simulink model "SixteenMuxInput"  (R2024b)
settings: Solver=VariableStepAuto  StartTime=0.0  StopTime=10.0  RelTol=1e-3
settings Model: Creator=ferbe  LastModifiedBy=ferbe

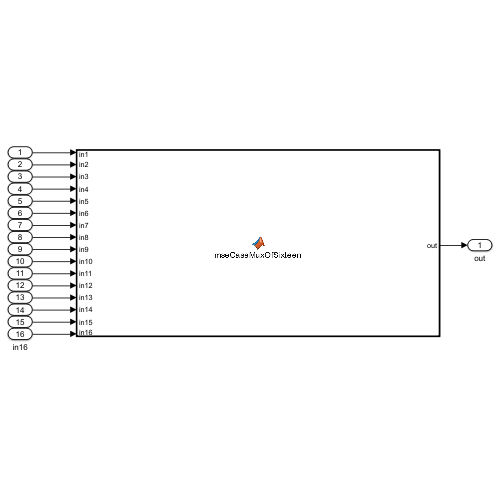
[thumbnail: Simulink's stored preview of the top-level diagram]
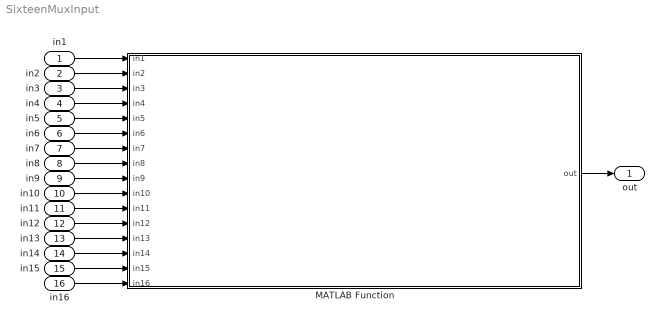
== system SixteenMuxInput ==
  in1 : Inport
  in2 : Inport  Port=2
  in3 : Inport  Port=3
  in4 : Inport  Port=4
  in5 : Inport  Port=5
  in6 : Inport  Port=6
  in7 : Inport  Port=7
  in8 : Inport  Port=8
  in9 : Inport  Port=9
  in10 : Inport  Port=10
  in11 : Inport  Port=11
  in12 : Inport  Port=12
  in13 : Inport  Port=13
  in14 : Inport  Port=14
  in15 : Inport  Port=15
  in16 : Inport  Port=16
  MATLAB Function : MATLAB Function  TreatAsAtomicUnit=on
  out : Outport
  wires:
  in1/1 -> MATLAB Function/1(in1)
  in2/1 -> MATLAB Function/2(in2)
  in3/1 -> MATLAB Function/3(in3)
  in4/1 -> MATLAB Function/4(in4)
  in5/1 -> MATLAB Function/5(in5)
  in6/1 -> MATLAB Function/6(in6)
  in7/1 -> MATLAB Function/7(in7)
  in8/1 -> MATLAB Function/8(in8)
  in9/1 -> MATLAB Function/9(in9)
  in10/1 -> MATLAB Function/10(in10)
  in11/1 -> MATLAB Function/11(in11)
  in12/1 -> MATLAB Function/12(in12)
  in13/1 -> MATLAB Function/13(in13)
  in14/1 -> MATLAB Function/14(in14)
  in15/1 -> MATLAB Function/15(in15)
  in16/1 -> MATLAB Function/16(in16)
  MATLAB Function/1(out) -> out/1

== matlab function SixteenMuxInput/MATLAB Function ==
  data: in1 input; out output; in2 input; in3 input; in4 input; in5 input; in6 input; in7 input; in8 input; in9 input; in10 input; in11 input; in12 input; in13 input; in14 input; in15 input; in16 input
function out = mseCaseMuxOfSixteen(in1, in2, in3, in4, in5, in6, in7, in8, in9, in10, in11, in12, in13, in14, in15, in16)
% Method to mux 16 inputs into one of 16 possible outputs based on
% the first non-negative input.  To be paired with CaseSplitOfFour.
%
% Written by: Darian Muresan
% Last Modified: 10/10/2024

% Handle missing inputs
if nargin < 2
    in2 = -1;
    in3 = -1;
    in4 = -1;
    in5 = -1;
    in6 = -1;
    in7 = -1;
    in8 = -1;
    in9 = -1;
    in10 = -1;
    in11 = -1;
    in12 = -1;
    in13 = -1;
    in14 = -1;
    in15 = -1;
    in16 = -1;
elseif nargin < 3
    in3 = -1;
    in4 = -1;
    in5 = -1;
    in6 = -1;
    in7 = -1;
    in8 = -1;
    in9 = -1;
    in10 = -1;
    in11 = -1;
    in12 = -1;
    in13 = -1;
    in14 = -1;
    in15 = -1;
    in16 = -1;
elseif nargin < 4
    in4 = -1;
    in5 = -1;
    in6 = -1;
    in7 = -1;
    in8 = -1;
    in9 = -1;
    in10 = -1;
    in11 = -1;
    in12 = -1;
    in13 = -1;
    in14 = -1;
    in15 = -1;
    in16 = -1;
elseif nargin < 5
    in5 = -1;
    in6 = -1;
    in7 = -1;
    in8 = -1;
    in9 = -1;
    in10 = -1;
    in11 = -1;
    in12 = -1;
    in13 = -1;
    in14 = -1;
    in15 = -1;
    in16 = -1;
elseif nargin < 6
    in6 = -1;
    in7 = -1;
    in8 = -1;
    in9 = -1;
    in10 = -1;
    in11 = -1;
    in12 = -1;
    in13 = -1;
    in14 = -1;
    in15 = -1;
    in16 = -1;
elseif nargin < 7
    in7 = -1;
    in8 = -1;
    in9 = -1;
    in10 = -1;
    in11 = -1;
    in12 = -1;
    in13 = -1;
    in14 = -1;
    in15 = -1;
    in16 = -1;
elseif nargin < 8
    in8 = -1;
    in9 = -1;
    in10 = -1;
    in11 = -1;
    in12 = -1;
    in13 = -1;
    in14 = -1;
    in15 = -1;
    in16 = -1;
elseif nargin < 9
    in9 = -1;
    in10 = -1;
    in11 = -1;
    in12 = -1;
    in13 = -1;
    in14 = -1;
    in15 = -1;
    in16 = -1;
elseif nargin < 10
    in10 = -1;
    in11 = -1;
    in12 = -1;
    in13 = -1;
    in14 = -1;
    in15 = -1;
    in16 = -1;
elseif nargin < 11
    in11 = -1;
    in12 = -1;
    in13 = -1;
    in14 = -1;
    in15 = -1;
    in16 = -1;
elseif nargin < 12
    in12 = -1;
    in13 = -1;
    in14 = -1;
    in15 = -1;
    in16 = -1;
elseif nargin < 13
    in13 = -1;
    in14 = -1;
    in15 = -1;
    in16 = -1;
elseif nargin < 14
    in14 = -1;
    in15 = -1;
    in16 = -1;
elseif nargin < 15
    in15 = -1;
    in16 = -1;
elseif nargin < 16
    in16 = -1;
end

% Select the first non-negative input
if in1 >= 0
    out = in1;
elseif in2 >= 0
    out = in2;
elseif in3 >= 0
    out = in3;
elseif in4 >= 0
    out = in4;
elseif in5 >= 0
    out = in5;
elseif in6 >= 0
    out = in6;
elseif in7 >= 0
    out = in7;
elseif in8 >= 0
    out = in8;
elseif in9 >= 0
    out = in9;
elseif in10 >= 0
    out = in10;
elseif in11 >= 0
    out = in11;
elseif in12 >= 0
    out = in12;
elseif in13 >= 0
    out = in13;
elseif in14 >= 0
    out = in14;
elseif in15 >= 0
    out = in15;
elseif in16 >= 0
    out = in16;
else
    out = -1;
end
